simulink model "SummaLab"  (Simulink 4.00)
settings: Solver=ode45  StartTime=0.0  StopTime=10.0  RelTol=1e-3
settings Model: LastModifiedBy=user

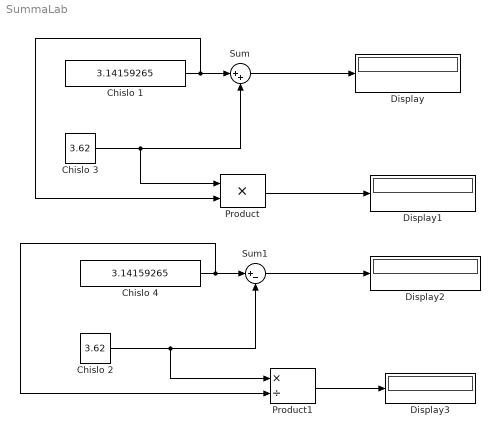
== system SummaLab ==
  Chislo 1 : Constant  Value=3.14159265
  Chislo 2 : Constant  Value=3.62
  Chislo 3 : Constant  Value=3.62
  Chislo 4 : Constant  Value=3.14159265
  Display{,1..3} (4 alike) : Display
      Display1 settings: Format=short
      Display3 settings: Format=short
  Product : Product  Inputs=2  Multiplication=Element-wise(.*)  SaturateOnIntegerOverflow=on
  Product1 : Product  Inputs=*/  Multiplication=Element-wise(.*)  SaturateOnIntegerOverflow=on
  Sum : Sum  Inputs=|++  SaturateOnIntegerOverflow=on
  Sum1 : Sum  Inputs=|+-  SaturateOnIntegerOverflow=on
  wires:
  Chislo 3/1 -> Sum/2, Product/1
  Chislo 1/1 -> Sum/1, Product/2
  Product/1 -> Display1/1
  Sum/1 -> Display/1
  Chislo 2/1 -> Sum1/2, Product1/1
  Chislo 4/1 -> Sum1/1, Product1/2
  Sum1/1 -> Display2/1
  Product1/1 -> Display3/1
